simulink model "CiEngineCore"  (R2017b)
settings: Solver=VariableStepAuto  StartTime=0.0  StopTime=inf  RelTol=1e-3  EnableMultiTasking=on
model workspace (MAT data in the model file):
  AFRStoich = 14.6
  AirFilterArea = 0.000962112750162
  AirIntakeVol = 0.0018
  C_eng = 40000
  CompEff = [0.2 0.2 0.2 0.2 0.2 0.2 0.2 0.2 0.2 0.2 0.2 0.2 ... (6000 elements, 60x100)]
  CompMassFlwRate = [0 0.00256701884694 0.00511455880808 0.00766649491749 0.0102195028494 0.0127729401774 0.0153265889731 0.017880362476 0.0204342099213 0.0229881081418 0.0255420430633 0.0280960028754 ... (6000 elements, 60x100)]
  CompPrsRatioBreakPoints = [1 1.02808080808 1.05616161616 1.08424242424 1.11232323232 1.1404040404 1.16848484848 1.19656565657 1.22464646465 1.25272727273 1.28080808081 1.30888888889 ... (100 elements, 1x100)]
  CompRefPrs = 101325
  CompRefTemp = 300
  CompSpdBreakPoints = [0 422.344846438 844.689692876 1267.03447648 1689.3794067 2111.72412747 2534.06895296 2956.4139879 3378.75881339 3801.10374361 4223.44825494 4645.79349931 ... (60 elements, 1x60)]
  CoolantTemp = 310
  Cps = 2
  EgrArea = 0.000314159265359
  EgrCoolantTemp = 360
  EgrEffectiveness = 0.8
  ExhSysArea = 0.000804247719319
  ExhSysVol = 0.0008
  IcEffectiveness = 0.9
  InjSlp = 6.45161290323
  LHV = 47300000
  NCyl = 4
  Pstd = 101325
  Rair = 287.05
  Rexh = 297
  T_cool_start = 355
  T_coolnt_init = 355
  T_coolnt_max = 375
  Tstd = 293.15
  TurbEff = [0.008 0.008 0.008 0.008 0.008 0.008 0.008 0.008 0.008 0.008 0.008 0.008 ... (28800 elements, 60x80x6)]
  TurbMassFlwRate = [7.02000192308e-05 7.02000192308e-05 7.02000192308e-05 7.02000192308e-05 7.02000192308e-05 7.02000192308e-05 7.02000192308e-05 7.02000192308e-05 7.02000192308e-05 7.02000192308e-05 7.02000192308e-05 7.02000192308e-05 ... (28800 elements, 60x80x6)]
  TurbPrsRatioBreakPoints = [1 1.03481012658 1.06962025316 1.10443037975 1.13924050633 1.17405063291 1.20886075949 1.24367088608 1.27848101266 1.31329113924 1.34810126582 1.38291139241 ... (80 elements, 1x80)]
  TurbRackBreakPoints = [0 0.2 0.3 0.5 0.7 1]
  TurbRefPrs = 101325
  TurbRefTemp = 300
  TurbSpdBreakPoints = [0 267.361773363 534.723546727 802.08532009 1069.44709345 1336.80886682 1604.17064018 1871.53241354 2138.89418691 2406.25596027 2673.61773363 2940.979507 ... (60 elements, 1x60)]
  TurboInertia = 6e-06
  Vd = 0.0015
  Vexh = 0.000696349540849
  Vint = 0.00286
  cp_air = 1005
  cp_exh = 1005
  f_co = [1.40212981041e-06 1.40212981041e-06 1.6332261526e-06 1.85316257772e-06 2.13933731744e-06 2.5578774362e-06 3.5801963158e-06 5.71066968323e-06 9.06691784867e-06 1.17856264254e-05 1.13266430068e-05 1.17075290539e-05 ... (240 elements, 16x15)]
  f_co2 = [0.0565058276487 0.0565058276487 0.0680775298139 0.0795416117649 0.0927502758383 0.108898516704 0.135970777083 0.163224038089 0.18390566243 0.187824483941 0.180854201863 0.181624048607 ... (240 elements, 16x15)]
  f_exhfrac_n_bpt = [750 1053.57142857 1357.14285714 1660.71428571 1964.28571429 2267.85714286 2571.42857143 2875 3178.57142857 3482.14285714 3785.71428571 4089.28571429 ... (15 elements, 1x15)]
  f_exhfrac_trq_bpt = [0 15 26.4285714286 37.8571428571 49.2857142857 60.7142857143 72.1428571429 83.5714285714 95 106.428571429 117.857142857 129.285714286 ... (16 elements, 1x16)]
  f_fric_temp_bpt = [274 276 278 280 282 284 286 288 290 292 294 296 ... (54 elements, 1x54)]
  f_fric_temp_mod = [3.96 3.22 2.56 2.26 2.11 2 1.9 1.83 1.76 1.7 1.65 1.6 ... (54 elements, 1x54)]
  f_hc = [1.08896576916e-07 1.08896576916e-07 1.53414498342e-07 2.00715453959e-07 2.48790869997e-07 2.97869368014e-07 3.52504999231e-07 4.04349945817e-07 4.52780325277e-07 4.91342452993e-07 4.91996758973e-07 4.96487624267e-07 ... (240 elements, 16x15)]
  f_nox = [9.38886565825e-05 9.38886565825e-05 0.000158278744526 0.000381657424268 0.00062836202089 0.000865097048745 0.000965103000667 0.00083216127124 0.00082959112316 0.00143554359074 0.00196340813932 0.0020351396325 ... (240 elements, 16x15)]
  f_nv = [0.954646224834 0.927678310575 0.901063682417 0.875710037198 0.852450535311 0.831986822876 0.814844392337 0.80134438932 0.791593989181 0.785495277781 0.782770492696 0.782999798686 ... (450 elements, 30x15)]
  f_nv_n_bpt = [1000 1285.71428571 1571.42857143 1857.14285714 2142.85714286 2428.57142857 2714.28571429 3000 3285.71428571 3571.42857143 3857.14285714 4142.85714286 ... (15 elements, 1x15)]
  f_nv_prs_bpt = [95 100.344827586 105.689655172 111.034482759 116.379310345 121.724137931 127.068965517 132.413793103 137.75862069 143.103448276 148.448275862 153.793103448 ... (30 elements, 1x30)]
  f_t_exh = [358.711368346 429.963145924 497.987869771 559.016510887 625.497016294 690.207854611 731.780908025 749.899407528 764.155922317 789.797182974 824.513264157 858.92580636 ... (240 elements, 16x15)]
  f_t_exh_f_bpt = [0 3.57 6.855 10.14 13.425 16.71 19.995 23.28 26.565 29.85 33.135 36.42 ... (16 elements, 1x16)]
  f_t_exh_n_bpt = [1000 1285.71428571 1571.42857143 1857.14285714 2142.85714286 2428.57142857 2714.28571429 3000 3285.71428571 3571.42857143 3857.14285714 4142.85714286 ... (15 elements, 1x15)]
  f_tq_apc_bpt = [94.6146459029 109.976602506 125.338559109 140.700515712 156.062472315 171.424428919 186.786385522 202.148342125 217.510298728 232.872255331 248.234211934 263.596168537 ... (15 elements, 1x15)]
  f_tq_apc_mod = [0.999715885044 0.999538569407 0.999259905514 0.998809242093 0.998358578671 0.997880679846 0.997234389999 0.996588100153 0.995941810306 0.99547925674 0.995035391789 0.994591526839 ... (240 elements, 15x16)]
  f_tq_fric = [0 0 0 0 0 0 0 0 0 0 0 0 ... (256 elements, 16x16)]
  f_tq_inr = [0 18.932941535 39.3255223176 57.8807366655 73.6414164249 90.1575991353 102.879416349 112.92944314 130.905512841 149.615511709 168.234721026 187.879026911 ... (256 elements, 16x16)]
  f_tq_inr_f_bpt = [0 3.57 6.855 10.14 13.425 16.71 19.995 23.28 26.565 29.85 33.135 36.42 ... (16 elements, 1x16)]
  f_tq_inr_n_bpt = [0 1000 1285.71428571 1571.42857143 1857.14285714 2142.85714286 2428.57142857 2714.28571429 3000 3285.71428571 3571.42857143 3857.14285714 ... (16 elements, 1x16)]
  f_tq_mainsoi_bpt = [-15 -13.7142857143 -12.4285714286 -11.1428571429 -9.85714285714 -8.57142857143 -7.28571428571 -6 -4.71428571429 -3.42857142857 -2.14285714286 -0.857142857143 ... (15 elements, 1x15)]
  f_tq_mainsoi_mod = [0.81078150005 0.827839263513 0.848673573925 0.874587588348 0.900164013454 0.923298328972 0.948048831471 0.970618714872 0.98831830141 0.997452724955 1 1 ... (240 elements, 15x16)]
  f_tq_map_bpt = [94.6146459029 109.976602506 125.338559109 140.700515712 156.062472315 171.424428919 186.786385522 202.148342125 217.510298728 232.872255331 248.234211934 263.596168537 ... (15 elements, 1x15)]
  f_tq_map_mod = [0.882177094009 0.934851504719 0.96634483908 0.97127123182 0.962954413121 0.952665164101 0.94513861625 0.942129377179 0.94335561462 0.947447812134 0.952949052459 0.958725491494 ... (240 elements, 15x16)]
  f_tq_mat_bpt = [35 42.8571428571 50.7142857143 58.5714285714 66.4285714286 74.2857142857 82.1428571429 90 97.8571428571 105.714285714 113.571428571 121.428571429 ... (15 elements, 1x15)]
  f_tq_mat_mod = [0.979193935333 0.989700620258 0.997707737278 1 0.992841543128 0.973230182048 0.94195882355 0.902873432246 0.86074346216 0.81947608235 0.779242235611 0.739783745312 ... (240 elements, 15x16)]
  f_tq_nf = [nan nan nan nan nan nan nan nan nan nan nan nan ... (256 elements, 16x16)]
  f_tq_nf_f_bpt = [0 3.57 6.855 10.14 13.425 16.71 19.995 23.28 26.565 29.85 33.135 36.42 ... (16 elements, 1x16)]
  f_tq_nf_n_bpt = [0 1000 1285.71428571 1571.42857143 1857.14285714 2142.85714286 2428.57142857 2714.28571429 3000 3285.71428571 3571.42857143 3857.14285714 ... (16 elements, 1x16)]
  f_tq_pump = [0 0 0 0 0 0 0 0 0 0 0 0 ... (256 elements, 16x16)]
  tau_cool = 3000
undefined symbols (not defined in the file): ThrAngToC
libraries: autolibfundflw x11, autolibboost x3, autolibcoreeng x1, simulink x1
(part 2 of 2)

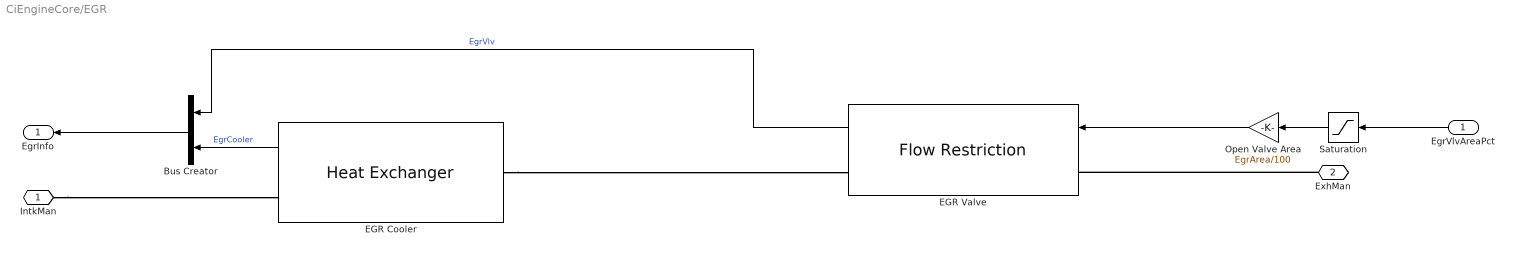
== system CiEngineCore/EGR ==
  EgrVlvAreaPct : Inport
  Bus Creator : BusCreator  Inputs=2
  EGR Cooler : autolibfundflw/Heat Exchanger  EffctModelPopup=Constant  CoolTempInputPopup=Constant  ImageTypePopup=EGR cooler  ep_cnst=EgrEffectiveness  T_cool_cnst=EgrCoolantTemp  cp=cp_exh
      settings: SourceProductName=Powertrain Blockset  SourceProductBaseCode=PW
  EGR Valve : autolibfundflw/Flow Restriction  AreaPopup=External input  ImageTypePopup=Hot  gamma=cp_exh / (cp_exh - Rexh)  R=Rair  Plim=0.9  Aorf_cnst=.1  Cd_cnst=1  Cd_ext=1  Dthr=ThrDiam  ThrCd=ThrAngToC(:,2)  ThrAngBpts=ThrAngToC(:,1)
      settings: SourceProductName=Powertrain Blockset  SourceProductBaseCode=PW
  Open Valve Area : Gain  Gain=EgrArea/100
  Saturation : Saturate  UpperLimit=100  LowerLimit=0
  IntkMan : PMIOPort  Port=1  Side=Right
  ExhMan : PMIOPort  Port=2  Side=Left
  EgrInfo : Outport
  wires:
  EgrVlvAreaPct/1 -> Saturation/1
  Open Valve Area/1 -> EGR Valve/1
  Saturation/1 -> Open Valve Area/1
  Bus Creator/1 -> EgrInfo/1
  EGR Cooler/1 -> Bus Creator/2  "EgrCooler"
  EGR Valve/1 -> Bus Creator/1  "EgrVlv"
  connections:
  EGR Cooler/LConn1 -- EGR Valve/RConn1
  IntkMan/RConn1 -- EGR Cooler/RConn1
  ExhMan/RConn1 -- EGR Valve/LConn1

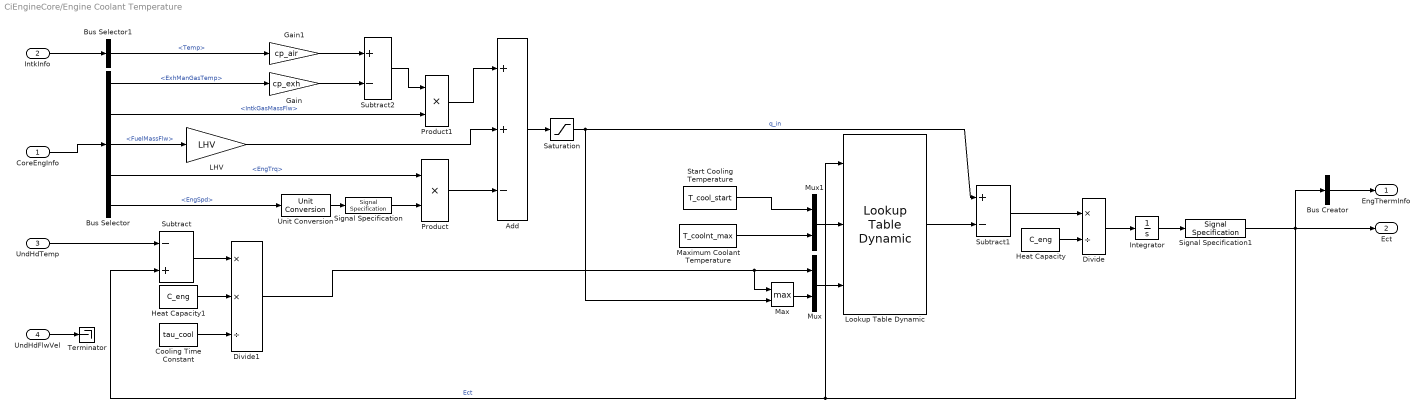
== system CiEngineCore/Engine Coolant Temperature ==
  CoreEngInfo : Inport
  IntkInfo : Inport  Port=2
  UndHdTemp : Inport  Port=3
  UndHdFlwVel : Inport  Port=4
  Add : Sum  Inputs=++-
  Bus Creator : BusCreator  Inputs=1
  Bus Selector : BusSelector  OutputSignals=ExhManGasTemp,IntkGasMassFlw,FuelMassFlw,EngTrq,EngSpd
  Bus Selector1 : BusSelector  OutputSignals=Vol.Temp
  Cooling Time Constant : Constant  Value=tau_cool
  Divide : Product  Inputs=*/
  Divide1 : Product  Inputs=**/
  Gain : Gain  Gain=cp_exh
  Gain1 : Gain  Gain=cp_air
  Heat Capacity : Constant  Value=C_eng
  Heat Capacity1 : Constant  Value=C_eng
  Integrator : Integrator  InitialCondition=T_coolnt_init  LimitOutput=on  UpperSaturationLimit=T_coolnt_max  LowerSaturationLimit=0  ZeroCross=off
  LHV : Gain  Gain=LHV
  Lookup Table Dynamic : simulink/Lookup Tables/Lookup Table Dynamic  LookUpMeth=Interpolation-Use End Values  OutDataType=fixdt('double')  OutScaling=[]  OutputDataTypeScalingMode=Specify via dialog  OutDataTypeStr=double  DoSatur=off
      settings: SourceProductName=Simulink
  Max : MinMax  Function=max  Inputs=2  ZeroCross=off
  Maximum Coolant Temperature : Constant  Value=T_coolnt_max
  Mux : Mux  Inputs=2
  Mux1 : Mux  Inputs=2
  Product : Product
  Product1 : Product
  Saturation : Saturate  UpperLimit=Inf  LowerLimit=0
  Signal Specification : SignalSpecification  Unit=rad/s
  Signal Specification1 : SignalSpecification  Unit=K
  Start Cooling Temperature : Constant  Value=T_cool_start
  Subtract : Sum  Inputs=-+
  Subtract1 : Sum  Inputs=+-
  Subtract2 : Sum  Inputs=+-
  Terminator : Terminator
  Unit Conversion : UnitConversion
  EngThermInfo : Outport  Unit=K
  Ect : Outport  Port=2  Unit=K
  wires:
  UndHdTemp/1 -> Subtract/1
  Heat Capacity/1 -> Divide/2
  Unit Conversion/1 -> Signal Specification/1
  Maximum Coolant Temperature/1 -> Mux1/2
  Signal Specification1/1 -> Subtract/2, Lookup Table Dynamic/1, Bus Creator/1, Ect/1  "Ect"
  UndHdFlwVel/1 -> Terminator/1
  Gain/1 -> Subtract2/2
  Bus Selector/4 -> Product/1  "<EngTrq>"
  Mux1/1 -> Lookup Table Dynamic/2
  Divide1/1 -> Max/1, Mux/1
  Heat Capacity1/1 -> Divide1/2
  Mux/1 -> Lookup Table Dynamic/3
  Start Cooling Temperature/1 -> Mux1/1
  Subtract/1 -> Divide1/1
  Saturation/1 -> Max/2, Subtract1/1  "q_in"
  Signal Specification/1 -> Product/2
  LHV/1 -> Add/2
  Product/1 -> Add/3
  Bus Selector/5 -> Unit Conversion/1  "<EngSpd>"
  Cooling Time Constant/1 -> Divide1/3
  CoreEngInfo/1 -> Bus Selector/1
  Bus Selector/3 -> LHV/1  "<FuelMassFlw>"
  Bus Selector/1 -> Gain/1  "<ExhManGasTemp>"
  Gain1/1 -> Subtract2/1
  Bus Selector1/1 -> Gain1/1  "<Temp>"
  Divide/1 -> Integrator/1
  Subtract1/1 -> Divide/1
  Lookup Table Dynamic/1 -> Subtract1/2
  Max/1 -> Mux/2
  Bus Creator/1 -> EngThermInfo/1
  IntkInfo/1 -> Bus Selector1/1
  Integrator/1 -> Signal Specification1/1
  Subtract2/1 -> Product1/1
  Bus Selector/2 -> Product1/2  "<IntkGasMassFlw>"
  Product1/1 -> Add/1
  Add/1 -> Saturation/1

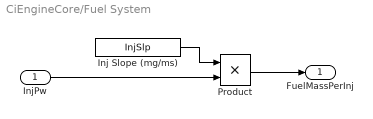
== system CiEngineCore/Fuel System ==
  InjPw : Inport
  Inj Slope (mg/ms) : Constant  Value=InjSlp
  Product : Product
  FuelMassPerInj : Outport
  wires:
  InjPw/1 -> Product/2
  Inj Slope (mg/ms)/1 -> Product/1
  Product/1 -> FuelMassPerInj/1

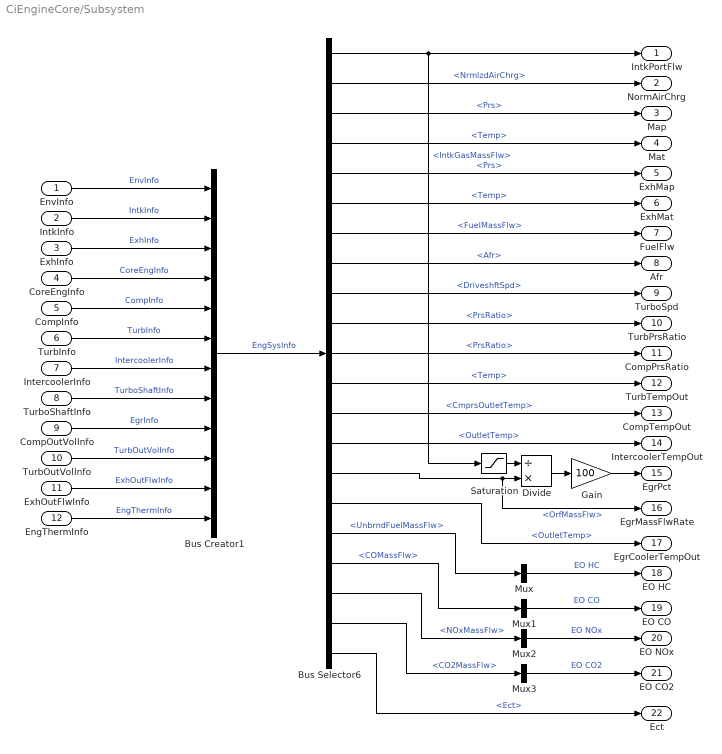
== system CiEngineCore/Subsystem ==
  EnvInfo : Inport
  IntkInfo : Inport  Port=2
  ExhInfo : Inport  Port=3
  CoreEngInfo : Inport  Port=4
  CompInfo : Inport  Port=5
  TurbInfo : Inport  Port=6
  IntercoolerInfo : Inport  Port=7
  TurboShaftInfo : Inport  Port=8
  CompOutVolInfo : Inport  Port=9
  TurbOutVolInfo : Inport  Port=10
  ExhOutFlwInfo : Inport  Port=11
  EngThermInfo : Inport  Port=12
  Bus Creator1 : BusCreator  Inputs=12
  Bus Selector6 : BusSelector  OutputSignals=CoreEngInfo.IntkGasMassFlw,CoreEngInfo.NrmlzdAirChrg,IntkInfo.Vol.Prs,IntkInfo.Vol.Temp,ExhInfo.Vol.Prs,ExhInfo.Vol.Temp,CoreEngInfo.FuelMassFlw,CoreEngInfo.Afr,TurboShaftInfo.DriveshftSpd,TurbInfo.PrsRatio,CompInfo.PrsRatio,TurbOutVolInfo.Vol.Temp,CompInfo.CmprsOutletTemp,IntercoolerInfo.OutletTemp,EgrInfo.EgrVlv.Flw.OrfMassFlw,EgrInfo.EgrCooler.OutletTemp,ExhOutFlwInfo.Flw.Species.UnbrndFuelMassFlw,ExhOutFlwInfo.Flw.Species.COMassFlw,ExhOutFlwInfo.Flw.Species.NOxMassFlw,ExhOutFlwInfo.Flw.Species.CO2MassFlw,EngThermInfo.Ect
  Divide : Product  Inputs=/*
  Gain : Gain  Gain=100
  Mux{,1..3} (4 alike) : Mux  Inputs=1
  Saturation : Saturate  UpperLimit=inf  LowerLimit=1e-6
  IntkPortFlw : Outport
  NormAirChrg : Outport  Port=2  Unit=1
  Map : Outport  Port=3
  Mat : Outport  Port=4
  ExhMap : Outport  Port=5
  ExhMat : Outport  Port=6
  FuelFlw : Outport  Port=7
  Afr : Outport  Port=8  Unit=1
  TurboSpd : Outport  Port=9
  TurbPrsRatio : Outport  Port=10
  CompPrsRatio : Outport  Port=11
  TurbTempOut : Outport  Port=12
  CompTempOut : Outport  Port=13
  IntercoolerTempOut : Outport  Port=14
  EgrPct : Outport  Port=15  Unit=%
  EgrMassFlwRate : Outport  Port=16
  EgrCoolerTempOut : Outport  Port=17
  EO HC : Outport  Port=18
  EO CO : Outport  Port=19
  EO NOx : Outport  Port=20
  EO CO2 : Outport  Port=21
  Ect : Outport  Port=22
  wires:
  TurbOutVolInfo/1 -> Bus Creator1/10  "TurbOutVolInfo"
  CompOutVolInfo/1 -> Bus Creator1/9  "EgrInfo"
  Bus Selector6/14 -> IntercoolerTempOut/1  "<OutletTemp>"
  Bus Selector6/13 -> CompTempOut/1  "<CmprsOutletTemp>"
  Bus Selector6/12 -> TurbTempOut/1  "<Temp>"
  Bus Selector6/11 -> CompPrsRatio/1  "<PrsRatio>"
  Bus Selector6/10 -> TurbPrsRatio/1  "<PrsRatio>"
  Bus Selector6/2 -> NormAirChrg/1  "<NrmlzdAirChrg>"
  Bus Selector6/8 -> Afr/1  "<Afr>"
  Bus Selector6/7 -> FuelFlw/1  "<FuelMassFlw>"
  Bus Selector6/6 -> ExhMat/1  "<Temp>"
  Bus Selector6/5 -> ExhMap/1  "<Prs>"
  Bus Selector6/4 -> Mat/1  "<Temp>"
  Bus Selector6/3 -> Map/1  "<Prs>"
  Bus Selector6/1 -> IntkPortFlw/1, Saturation/1  "<IntkGasMassFlw>"
  TurboShaftInfo/1 -> Bus Creator1/8  "TurboShaftInfo"
  TurbInfo/1 -> Bus Creator1/6  "TurbInfo"
  IntercoolerInfo/1 -> Bus Creator1/7  "IntercoolerInfo"
  Bus Creator1/1 -> Bus Selector6/1  "EngSysInfo"
  EnvInfo/1 -> Bus Creator1/1  "EnvInfo"
  CoreEngInfo/1 -> Bus Creator1/4  "CoreEngInfo"
  ExhInfo/1 -> Bus Creator1/3  "ExhInfo"
  IntkInfo/1 -> Bus Creator1/2  "IntkInfo"
  CompInfo/1 -> Bus Creator1/5  "CompInfo"
  Bus Selector6/15 -> Divide/2, EgrMassFlwRate/1  "<OrfMassFlw>"
  Bus Selector6/16 -> EgrCoolerTempOut/1  "<OutletTemp>"
  Divide/1 -> Gain/1
  Saturation/1 -> Divide/1
  Gain/1 -> EgrPct/1
  ExhOutFlwInfo/1 -> Bus Creator1/11  "ExhOutFlwInfo"
  Bus Selector6/17 -> Mux/1  "<UnbrndFuelMassFlw>"
  Bus Selector6/18 -> Mux1/1  "<COMassFlw>"
  Bus Selector6/19 -> Mux2/1  "<NOxMassFlw>"
  Bus Selector6/20 -> Mux3/1  "<CO2MassFlw>"
  Mux/1 -> EO HC/1  "EO HC"
  Mux1/1 -> EO CO/1  "EO CO"
  Mux2/1 -> EO NOx/1  "EO NOx"
  Mux3/1 -> EO CO2/1  "EO CO2"
  Bus Selector6/9 -> TurboSpd/1  "<DriveshftSpd>"
  Bus Selector6/21 -> Ect/1  "<Ect>"
  EngThermInfo/1 -> Bus Creator1/12  "EngThermInfo"
